simulink model "RLBicycleSimulinkModel"  (R2020a)
settings: Solver=VariableStepAuto  StartTime=0.0  StopTime=10000  RelTol=1e-3
PostLoadFcn:
  | set_param(gcs, 'ForceConsistencyChecking', 'off');
model workspace (MAT data in the model file):
  Sig = Simulink.Signal
  Sig.DataType = 'auto'
  Sig.Dimensions = -1
  Sig.DimensionsMode = 'auto'
  Sig.Complexity = 'auto'
  Sig.SampleTime = -1
  Sig.SamplingMode = 'auto'
undefined symbols (not defined in the file): QCarMap
libraries: robotmobilelib x1, rllib x1
settings Model: OrderedModelArguments=off  Creator=The MathWorks, Inc.  LastModifiedBy=guyot
settings DebuggingCC: SymbolicDimsDataTypeCodeGenerationDiagnostic=none

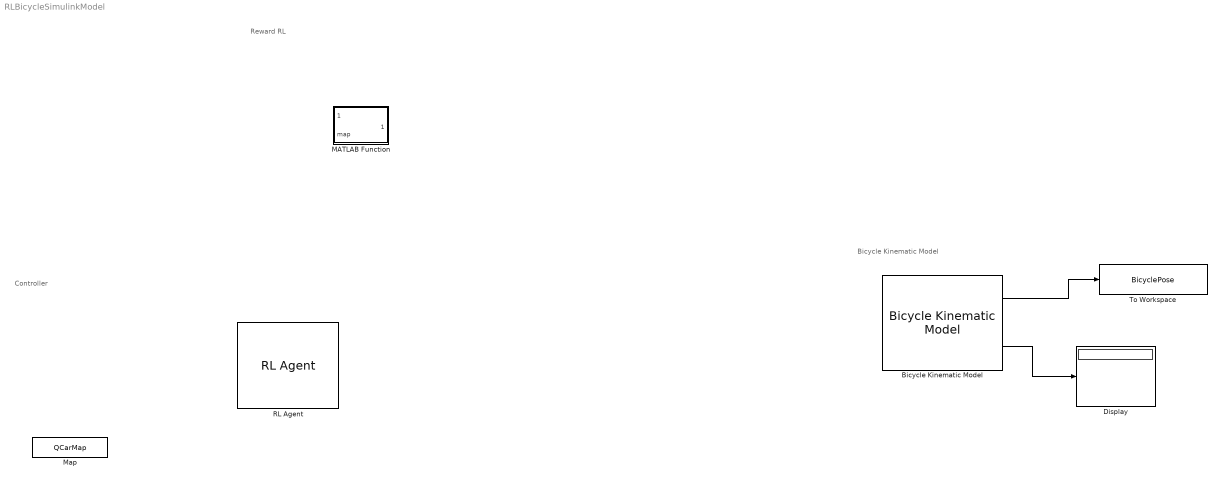
== system RLBicycleSimulinkModel ==
  note: Reward RL
  note: Bicycle Kinematic Model
  note: Controller
  Bicycle Kinematic Model : robotmobilelib/Bicycle Kinematic Model  VehicleInputs=Vehicle Speed & Heading Angular Velocity  WheelBase=0.5  VehicleSpeedRange=[-1 1]  MaxSteeringAngle=pi/3  InitialState=initialBicycle  SimulateUsing=Interpreted execution
      settings: SourceProductBaseCode=RO
  Display : Display
  MATLAB Function : MATLAB Function  TreatAsAtomicUnit=on
  Map : Constant  Value=QCarMap
  RL Agent : rllib/RL Agent  Agent=agentObj  ProvideReward=on  ProvideIsDone=on  ProvideCumRwd=off  TreatAsDirectFeedthrough=on  CollectLoggedSignals=on  CollectModelStates=on
  To Workspace : ToWorkspace  VariableName=BicyclePose  SampleTime=-1
  wires:
  Bicycle Kinematic Model/1 -> To Workspace/1
  Bicycle Kinematic Model/2 -> Display/1

== matlab function RLBicycleSimulinkModel/MATLAB Function ==
  data: bot_pos input; distMin output; map input
function distMin = distanceMin(bot_pos, map)
    distMin = 0;
